simulink model "pwpf"  (R2021b)
settings: Solver=VariableStepAuto  StartTime=0.0  StopTime=t_sim  RelTol=1e-3
values from neighbouring files (symbols this model uses):
  Km = inputArg(2)    [cost_pwpf.m]
  Tm = inputArg(1)    [cost_pwpf.m]
  u_off = inputArg(4)    [cost_pwpf.m]    (also in cost_pwpf_dis.m)
  u_on = h+u_off    [cost_pwpf.m]    (also in cost_pwpf_dis.m)
undefined symbols (not defined in the file or in its folder): min_on_off_time, test_freq, Thrust_analog
settings Model: Creator=Mehdi  LastModifiedBy=Mehdi
settings SolverCC: ZeroCrossAlgorithm=Adaptive  AlgebraicLoopSolver=TrustRegion
settings DebuggingCC: IgnoredZcDiagnostic=none  SFMachineParentedDataDiag=warning

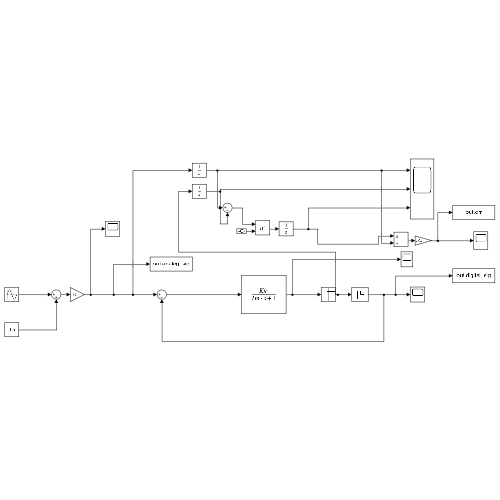
[thumbnail: Simulink's stored preview of the top-level diagram]
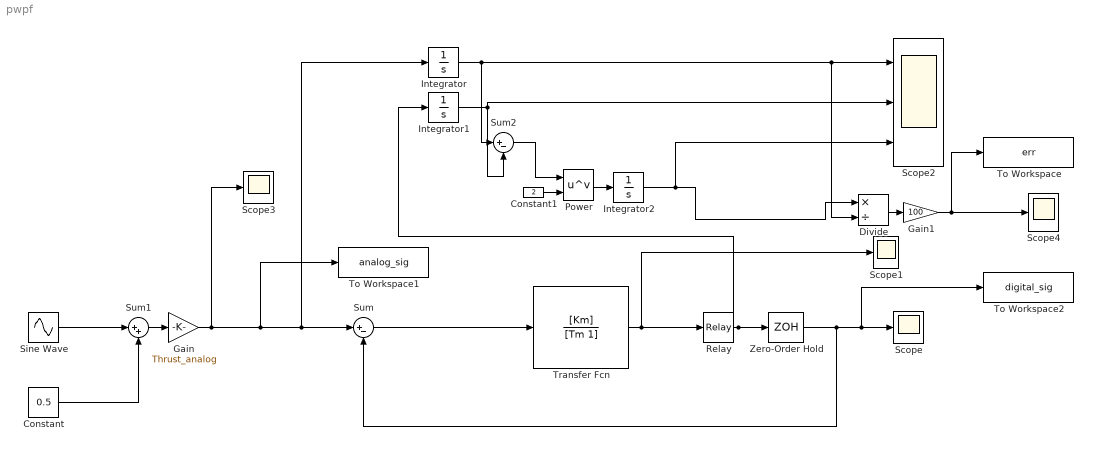
== system pwpf ==
  Constant : Constant  Value=0.5  VectorParams1D=off
  Constant1 : Constant  Value=2  VectorParams1D=off
  Divide : Product  Inputs=*/
  Gain : Gain  Gain=Thrust_analog
  Gain1 : Gain  Gain=100
  Integrator : Integrator
  Integrator1 : Integrator
  Integrator2 : Integrator
  Power : Math  Operator=pow  SaturateOnIntegerOverflow=on
  Relay : Relay  OnSwitchValue=u_on  OffSwitchValue=u_off  OnOutputValue=Thrust_digital
  Scope{,1,3..4} (4 alike) : Scope
  Scope2 : Scope  NumInputPorts=3
  Sine Wave : Sin  Amplitude=0.5  Frequency=test_freq  SampleTime=0
  Sum : Sum  Inputs=|+-
  Sum1 : Sum  Inputs=|++
  Sum2 : Sum  Inputs=|+-
  To Workspace : ToWorkspace  VariableName=err  SaveFormat=Timeseries  SampleTime=-1
      settings: MaxDataPoints=1
  To Workspace1 : ToWorkspace  VariableName=analog_sig  SaveFormat=Timeseries  SampleTime=-1
  To Workspace2 : ToWorkspace  VariableName=digital_sig  SaveFormat=Timeseries  SampleTime=-1
  Transfer Fcn : TransferFcn  Numerator=[Km]  Denominator=[Tm 1]
  Zero-Order Hold : ZeroOrderHold  SampleTime=min_on_off_time
  wires:
  Relay/1 -> Zero-Order Hold/1, Integrator1/1
  Transfer Fcn/1 -> Relay/1, Scope1/1
  Sum1/1 -> Gain/1
  Sum/1 -> Transfer Fcn/1
  Integrator/1 -> Sum2/1, Divide/2, Scope2/1
  Integrator1/1 -> Sum2/2, Scope2/2
  Sine Wave/1 -> Sum1/1
  Sum2/1 -> Power/1
  Gain/1 -> Scope3/1, To Workspace1/1, Integrator/1, Sum/1
  Constant/1 -> Sum1/2
  Power/1 -> Integrator2/1
  Integrator2/1 -> Scope2/3, Divide/1
  Constant1/1 -> Power/2
  Zero-Order Hold/1 -> Sum/2, To Workspace2/1, Scope/1
  Divide/1 -> Gain1/1
  Gain1/1 -> To Workspace/1, Scope4/1
